simulink model "telecom system"  (R2021b)
settings: Solver=VariableStepAuto  StartTime=0.0  StopTime=5e-3  MaxStep=1.0E-5  RelTol=1e-3
undefined symbols (not defined in the file or in its folder): max_time
libraries: simulink x4, dspstat3 x1, dspsrcs4 x1, dspsigops x1, dspspect3 x1
(part 1 of 3)
settings Model: Creator=A  LastModifiedBy=Shahryar
settings SolverCC: AlgebraicLoopSolver=TrustRegion
settings DebuggingCC: SFMachineParentedDataDiag=warning

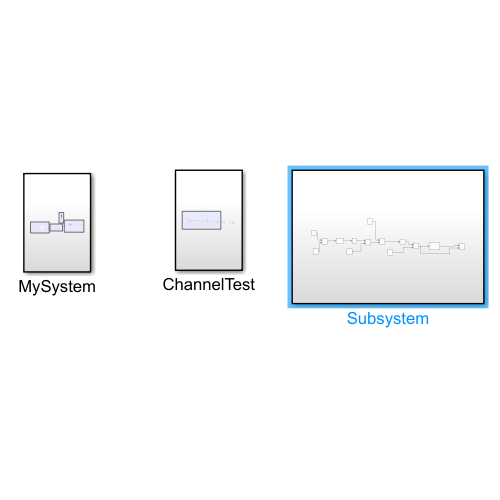
[thumbnail: Simulink's stored preview of the top-level diagram]
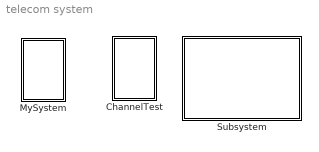
== system telecom system ==
  ChannelTest : Subsystem
  MySystem : Subsystem
  Subsystem : Subsystem

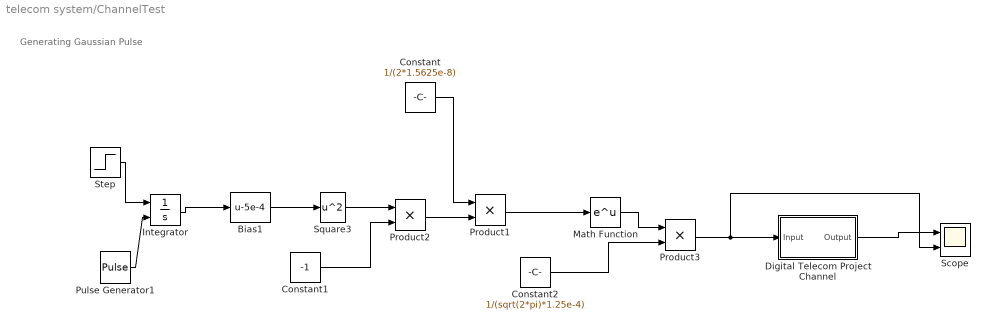
== system telecom system/ChannelTest ==
  note: Generating Gaussian Pulse
  Bias1 : Bias  Bias=-5e-4
  Constant : Constant  Value=1/(2*1.5625e-8)
  Constant1 : Constant  Value=-1  VectorParams1D=off
  Constant2 : Constant  Value=1/(sqrt(2*pi)*1.25e-4)
  Digital Telecom Project Channel : Subsystem  Tag=FilterWizardSubSystem
      settings: ErrorFcn=dspFilterRealizedInBasicElemsAlgLoopErrFcnCallback
  Integrator : Integrator  ExternalReset=rising
  Math Function : Math  SaturateOnIntegerOverflow=on
  Product1 : Product
  Product2 : Product
  Product3 : Product
  Pulse Generator1 : DiscretePulseGenerator  PulseType=Time based  Period=1e-3  PulseWidth=50
  Scope : Scope  NumInputPorts=2
  Square3 : Math  Operator=square  SaturateOnIntegerOverflow=on
  Step : Step  Time=1e-3  SampleTime=0
  wires:
  Integrator/1 -> Bias1/1
  Square3/1 -> Product2/1
  Bias1/1 -> Square3/1
  Product2/1 -> Product1/2
  Pulse Generator1/1 -> Integrator/2
  Constant1/1 -> Product2/2
  Constant/1 -> Product1/1
  Step/1 -> Integrator/1
  Product1/1 -> Math Function/1
  Math Function/1 -> Product3/1
  Constant2/1 -> Product3/2
  Product3/1 -> Scope/2, Digital Telecom Project Channel/1(Input)
  Digital Telecom Project Channel/1(Output) -> Scope/1

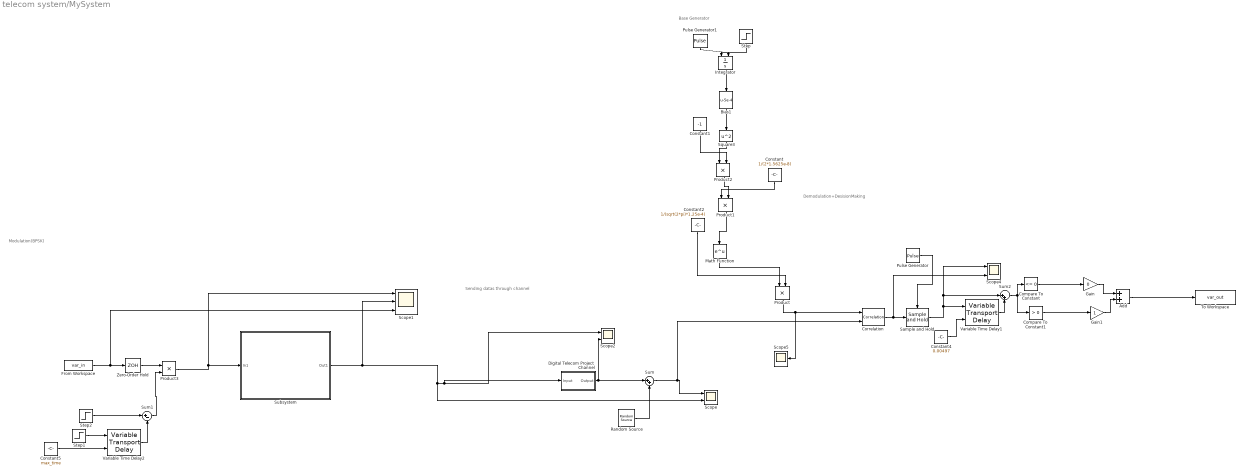
== system telecom system/MySystem ==
  note: Sending datas through channel
  note: Base Generator
  note: Demodulation+DesisionMaking
  note: Modulation(BPSK)
  Add : Sum
  Bias1 : Bias  Bias=-5e-4
  Compare To Constant : simulink/Logic and Bit Operations/Compare To Constant  relop=<=  const=0  OutDataTypeStr=boolean
  Compare To Constant1 : simulink/Logic and Bit Operations/Compare To Constant  relop=>  const=0  OutDataTypeStr=boolean
  Constant : Constant  Value=1/(2*1.5625e-8)
  Constant1 : Constant  Value=-1  VectorParams1D=off
  Constant2 : Constant  Value=1/(sqrt(2*pi)*1.25e-4)
  Constant4 : Constant  Value=0.00497
  Constant5 : Constant  Value=max_time
  Correlation : dspstat3/Correlation  domain=Time  roundingMode=Floor  overflowMode=off  outputDataTypeStr=Inherit: Same as accumulator  outputMin=[]  outputMax=[]  outputLastDataTypeStr=Inherit: Same as accumulator
      settings: SourceProductBaseCode=DS
  Digital Telecom Project Channel : Subsystem  Tag=FilterWizardSubSystem
      settings: ErrorFcn=dspFilterRealizedInBasicElemsAlgLoopErrFcnCallback
  From Workspace : FromWorkspace  VariableName=var_in  SampleTime=1e-3
  Gain : Gain  Gain=0
  Gain1 : Gain
  Integrator : Integrator  ExternalReset=rising
  Math Function : Math  SaturateOnIntegerOverflow=on
  Product{,1..3} (4 alike) : Product
  Pulse Generator : DiscretePulseGenerator  PulseType=Time based  Period=5e-4  PulseWidth=50
  Pulse Generator1 : DiscretePulseGenerator  PulseType=Time based  Period=1e-3  PulseWidth=50
  Random Source : dspsrcs4/Random Source  SrcType=Gaussian  NormMethod=Ziggurat  CltLength=12  MinVal=0  MaxVal=1  MeanVal=0  VarVal=5.4  RepMode=Not repeatable  rawSeed=1  IsInherit=off  SampMode=Discrete  SampTime=1e-3  SampFrame=1  DataType=Double  OutComplex=Real  OutputFrames=off
  Sample and Hold : dspsigops/Sample and Hold  trig=Rising edge  initCond=0  latchinput=off
  Scope : Scope  NumInputPorts=2
  Scope1 : Scope  NumInputPorts=3
  Scope2 : Scope  NumInputPorts=2
  Scope4 : Scope  NumInputPorts=2
  Scope5 : Scope
  Square3 : Math  Operator=square  SaturateOnIntegerOverflow=on
  Step : Step  Time=1e-3  SampleTime=0
  Step1 : Step  Time=0  SampleTime=0
  Step2 : Step  Time=0  SampleTime=0
  Subsystem : Subsystem
  Sum : Sum  Inputs=|++
  Sum1 : Sum  Inputs=|+-
  Sum2 : Sum  Inputs=|++
  To Workspace : ToWorkspace  VariableName=var_out  SampleTime=1e-3
      settings: Save2DSignal=2-D array (concatenate along first dimension)
  Variable Time Delay1 : VariableTransportDelay  MaximumDelay=10  MaximumPoints=4096
  Variable Time Delay2 : VariableTransportDelay  MaximumDelay=50000  MaximumPoints=4096
  Zero-Order Hold : ZeroOrderHold  SampleTime=1e-3
  wires:
  Product/1 -> Scope5/1, Correlation/1
  Random Source/1 -> Sum/2
  Step1/1 -> Variable Time Delay2/1
  Subsystem/1(Out1) -> Scope2/1, Digital Telecom Project Channel/1(Input), Scope/2, Scope1/2
  Product3/1 -> Subsystem/1(In1), Scope1/1
  From Workspace/1 -> Scope1/3, Zero-Order Hold/1
  Add/1 -> To Workspace/1
  Math Function/1 -> Product/1
  Constant2/1 -> Product/2
  Pulse Generator/1 -> Sample and Hold/Trigger
  Sample and Hold/1 -> Variable Time Delay1/1, Sum2/1, Scope4/1
  Correlation/1 -> Scope4/2, Sample and Hold/1
  Constant5/1 -> Variable Time Delay2/2
  Zero-Order Hold/1 -> Product3/1
  Digital Telecom Project Channel/1(Output) -> Scope2/2, Sum/1
  Variable Time Delay2/1 -> Sum1/2
  Compare To Constant1/1 -> Gain1/1
  Sum1/1 -> Product3/2
  Gain1/1 -> Add/2
  Sum/1 -> Correlation/2, Scope/1
  Variable Time Delay1/1 -> Sum2/2
  Constant4/1 -> Variable Time Delay1/2
  Sum2/1 -> Compare To Constant/1, Compare To Constant1/1
  Compare To Constant/1 -> Gain/1
  Step2/1 -> Sum1/1
  Gain/1 -> Add/1
  Pulse Generator1/1 -> Integrator/2
  Step/1 -> Integrator/1
  Constant1/1 -> Product2/2
  Integrator/1 -> Bias1/1
  Constant/1 -> Product1/1
  Bias1/1 -> Square3/1
  Product2/1 -> Product1/2
  Square3/1 -> Product2/1
  Product1/1 -> Math Function/1

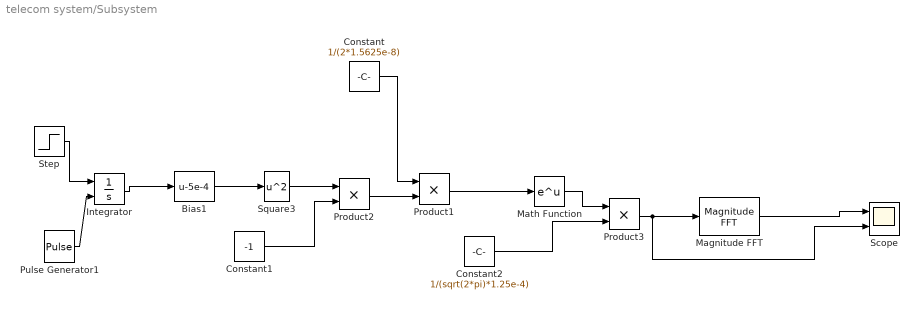
== system telecom system/Subsystem ==
  Bias1 : Bias  Bias=-5e-4
  Constant : Constant  Value=1/(2*1.5625e-8)
  Constant1 : Constant  Value=-1  VectorParams1D=off
  Constant2 : Constant  Value=1/(sqrt(2*pi)*1.25e-4)
  Integrator : Integrator  ExternalReset=rising
  Magnitude FFT : dspspect3/Magnitude FFT  mag_or_magsq=Magnitude  FFTImplementation=Auto  fftLenInherit=off  fftsize=256  WrapInput=on
      settings: SourceProductBaseCode=DS
  Math Function : Math  SaturateOnIntegerOverflow=on
  Product1 : Product
  Product2 : Product
  Product3 : Product
  Pulse Generator1 : DiscretePulseGenerator  PulseType=Time based  Period=1e-3  PulseWidth=50
  Scope : Scope  NumInputPorts=2
  Square3 : Math  Operator=square  SaturateOnIntegerOverflow=on
  Step : Step  Time=1e-3  SampleTime=0
  wires:
  Constant1/1 -> Product2/2
  Bias1/1 -> Square3/1
  Constant2/1 -> Product3/2
  Step/1 -> Integrator/1
  Constant/1 -> Product1/1
  Pulse Generator1/1 -> Integrator/2
  Integrator/1 -> Bias1/1
  Product2/1 -> Product1/2
  Math Function/1 -> Product3/1
  Product1/1 -> Math Function/1
  Square3/1 -> Product2/1
  Magnitude FFT/1 -> Scope/1
  Product3/1 -> Scope/2, Magnitude FFT/1
